simulink library "lib_wheel2"  (Simulink 4.1.1)
values from neighbouring files (symbols this model uses):
  logFlag = 1    [advSACompMaskInit.m]    (also in advSACompMaskInitR13.m)
undefined symbols (not defined in the file or in its folder): lib_help, NOTES, veh_air_density, veh_CD, veh_cg_height, veh_FA, veh_front_wt_frac, veh_gravity, veh_roadwheel_radius, veh_rr_a, veh_rr_alpha, veh_rr_b, veh_rr_beta, veh_rr_c, veh_wheelbase, wh_1st_rrc, wh_2nd_rrc, wh_axle_loss_mass, wh_axle_loss_trq, wh_fa_dl_brake_frac, wh_fa_dl_brake_mph, wh_fa_fric_brake_frac, wh_fa_fric_brake_mph, wh_front_active_bool, wh_inertia, wh_max_front_brake_force, wh_max_rear_brake_force, wh_pressure, wh_radius, wh_rear_active_bool, wh_slip, wh_slip_force_coeff
libraries: lib_wheel2 x61, lib_vehicle x2, lib_etc x2, lib_controls x2, lib_wheel x1
(part 1 of 14)
settings Model: LastModifiedBy=mokeefe
settings Model: ModifiedComment=|
  | mokeefe -- Thu Apr 18 08:40:34 2002 -- Version 1.10
  | saving the model:
  | o "without the model browser open"
  | o with only top-level screen visible
  | o with "fit to view" enabled
  | o with "status bar" off and "toolbar" off
  | o with "prompt to update model history with each save" on
settings Model: ModifiedHistory=|
  | mokeefe -- Thu Apr 18 08:40:34 2002 -- Version 1.10
  | saving the model:
  | o "without the model browser open"
  | o with only top-level screen visible
  | o with "fit to view" enabled
  | o with "status bar" off and "toolbar" off
  | o with "prompt to update model history with each save" on
  | 
  | mokeefe -- Thu Apr 18 08:40:34 2002 -- Version 1.10
  | saving the model:
  | o "without the model browser open"
  | o with only top-level screen visible
  | o with "fit to view" enabled
  | o with "status bar" off and "toolbar" off
  | o with "prompt to update model history with each save" on
  | 
  | ssprik -- Fri Feb 01 16:13:25 2002 -- Version 1.9
  | added wheel goto tag wh_trq_a
  | 
  | mokeefe -- Fri Jun 29 14:51:12 2001 -- Version 1.8
  | 
  | added sub-model component to calculate vehicle weight
  | 
  | mokeefe -- Fri Jun 29 14:49:48 2001 -- Version 1.7
  | 
  | 
  | mokeefe -- Thu Jun 28 14:08:49 2001 -- Version 1.6
  | 
  | replaced all 'veh_mass' references with a veh_mass plus a FROM block (originating from drive cycle) that gives variable cargo mass by time

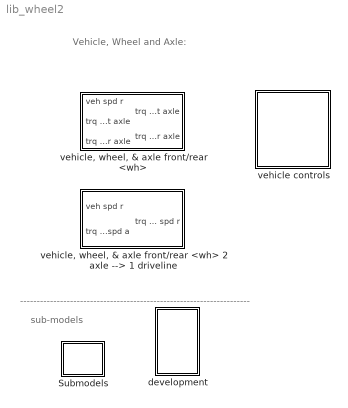
== system lib_wheel2 ==
  note: Vehicle, Wheel and Axle:
  note: ---------------------------------------------------------------------
  note: sub-models
  Submodels : Subsystem
      settings: RTWFcnNameOpts=Auto  RTWFileNameOpts=Auto
  development : Subsystem
      settings: RTWFcnNameOpts=Auto  RTWFileNameOpts=Auto
  vehicle controls : Subsystem
      settings: RTWFcnNameOpts=Auto  RTWFileNameOpts=Auto
  "vehicle, wheel, & axle front/rear <wh>" : Subsystem  mask(Stand-Alone Vehicle, Wheel, & Axle Mask){generalName='veh', generalName01='wh', logPick=Log, initFileName={}, modCell={}, imgFileName='bdi_wh&veh.jpg', DEBUG=OFF}
      mask prompts: generalName "General Name of Vehicle Component [char]"; generalName01 "General Name of Wheel Component [char]"; logPick "Log Variables to Workspace?"; initFileName "Initialization File(s) for VEH and WH [cell array of char]"; modCell "Modification Cell [2 column cell array of param and val]"; imgFileName "Icon image file name [char--evaluated]"
      mask init:
      | % initialization via m-file script
      | advSACompMaskInit;
      settings: RTWFcnNameOpts=Auto  RTWFileNameOpts=Auto
      mask StyleString: edit,edit,popup(Don't Log|Log),edit,edit,edit,popup(ON|OFF)
      mask Display: image(imread(imgFileName))
  "vehicle, wheel, & axle front/rear <wh> 2 axle --> 1 driveline" : Subsystem  mask(Stand-Alone Vehicle, Wheel, & Axle Mask){generalName='veh', generalName01='wh', logPick=Log, initFileName={}, modCell={}, imgFileName='bdi_wh&veh.jpg', DEBUG=OFF}
      mask prompts: generalName "General Name of Vehicle Component [char]"; generalName01 "General Name of Wheel Component [char]"; logPick "Log Variables to Workspace?"; initFileName "Initialization File(s) for VEH and WH [cell array of char]"; modCell "Modification Cell [2 column cell array of param and val]"; imgFileName "Icon image file name [char--evaluated]"
      mask init:
      | % initialization via m-file script
      | advSACompMaskInit;
      settings: RTWFcnNameOpts=Auto  RTWFileNameOpts=Auto
      mask StyleString: edit,edit,popup(Don't Log|Log),edit,edit,edit,popup(ON|OFF)
      mask Display: image(imread(imgFileName))

== system lib_wheel2/Submodels ==
  2 axle --> 1 driveline converter : Subsystem
      settings: RTWFcnNameOpts=Auto  RTWFileNameOpts=Auto
  braking strategy : Subsystem
      settings: RTWFcnNameOpts=Auto  RTWFileNameOpts=Auto
  config traction control : Subsystem  BlockChoice=traction control 2 axle
      settings: TemplateBlock=self  MemberBlocks=traction control 2 axle,traction control J2452 2 axle  RTWFcnNameOpts=Auto  RTWFileNameOpts=Auto
  current veh mass : Subsystem
      settings: RTWFcnNameOpts=Auto  RTWFileNameOpts=Auto
  force req'd to overcome rolling resistance (N) : Subsystem
      settings: RTWFcnNameOpts=Auto  RTWFileNameOpts=Auto
  force req'd to overcome rolling resistance (N) j2452 : Subsystem
      settings: RTWFcnNameOpts=Auto  RTWFileNameOpts=Auto
  front and rear brake controller (achievable) : Subsystem
      settings: RTWFcnNameOpts=Auto  RTWFileNameOpts=Auto
  rolling resistance force : Subsystem  BlockChoice=force req'd to overcome rolling resistance (N)
      settings: TemplateBlock=self  MemberBlocks=force req'd to overcome rolling resistance (N),force req'd to overcome rolling resistance (N) j2452  RTWFcnNameOpts=Auto  RTWFileNameOpts=Auto
  traction control 2 axle : Subsystem
      settings: RTWFcnNameOpts=Auto  RTWFileNameOpts=Auto
  traction control J2452 2 axle : Subsystem
      settings: RTWFcnNameOpts=Auto  RTWFileNameOpts=Auto
  vehicle speed : Subsystem  BlockChoice=vehicle speed (m/s)
      settings: TemplateBlock=self  MemberBlocks=vehicle speed (m/s),vehicle speed (m/s) j2452  RTWFcnNameOpts=Auto  RTWFileNameOpts=Auto
  vehicle speed (m/s) : Subsystem
      settings: RTWFcnNameOpts=Auto  RTWFileNameOpts=Auto
  vehicle speed (m/s) j2452 : Subsystem
      settings: RTWFcnNameOpts=Auto  RTWFileNameOpts=Auto

== system lib_wheel2/development ==
  wheel and axle  front/rear <wh> : Subsystem  mask(Stand-Alone Wheel/Axle Mask){generalName='wh', logPick=Log, initFileName={}, modCell={}, imgFileName='bdi_wh.jpg', DEBUG=OFF}
      mask prompts: generalName "General Name of this Component [char]"; logPick "Log Variables to Workspace?"; initFileName "Initialization File(s) [cell array of char]"; modCell "Modification Cell [2 column cell array of param and val]"; imgFileName "Icon image file name [char--evaluated]"
      mask init:
      | % initialization via m-file script
      | %advSACompMaskInit;
      settings: RTWFcnNameOpts=Auto  RTWFileNameOpts=Auto
      mask StyleString: edit,popup(Don't Log|Log),edit,edit,edit,popup(ON|OFF)
      mask Display: image(imread(imgFileName))
  wheel and axle  front/rear <wh> 2 axle --> 1 driveline : Subsystem
      settings: RTWFcnNameOpts=Auto  RTWFileNameOpts=Auto
      mask Display: image(imread('bdi_wh.jpg'))

== system lib_wheel2/vehicle controls ==
  Bus Selector : BusSelector  OutputSignals=signal1  MuxedOutput=off
  Bus Selector1 : BusSelector  OutputSignals=signal1  MuxedOutput=off
  Bus Selector2 : BusSelector  OutputSignals=signal1  MuxedOutput=off
  dummy controls : Subsystem
      settings: RTWFcnNameOpts=Auto  RTWFileNameOpts=Auto
  tag scope: vehControl=global
  wires:
  dummy controls/1(control sig) -> [vehControl]
  [Sensors] -> Bus Selector/1
  Bus Selector/1 -> dummy controls/1(initial vehicle velocity (m/s))  "<signal1>"
  Bus Selector1/1 -> dummy controls/2(vehicle's current mass (kg))  "<signal1>"
  Bus Selector2/1 -> dummy controls/3(current road grade)  "<signal1>"
  [Sensors] -> Bus Selector2/1
  [Sensors] -> Bus Selector1/1

== system lib_wheel2/vehicle, wheel, & axle front/rear <wh> ==
  note: Vehicle, Wheel, and Axle
  veh spd r : Inport  Port=1  LatchInput=off
  "trq & spd a, front axle" : Inport  Port=2  LatchInput=off
  "trq & spd a, rear axle" : Inport  Port=3  LatchInput=off
  models and interface : Subsystem
      settings: RTWFcnNameOpts=Auto  RTWFileNameOpts=Auto
  "trq & spd r, front axle" : Outport  Port=1  InitialOutput=0
  "trq & spd r, rear axle" : Outport  Port=2  InitialOutput=0
  tag scope: vehReqOut=global, vehSensors=global
  wires:
  veh spd r/1 -> models and interface/1(vehicle speed req'd at end of time step (m/s))
  "trq & spd a, front axle"/1 -> models and interface/2("torque and speed available from drivetrain into front axle (Nm), (rad/s)")
  "trq & spd a, rear axle"/1 -> models and interface/3("torque and speed available from drivetrain into rear axle (Nm), (rad/s)")
  [vehControl] -> models and interface/4(control)
  models and interface/1(requested out) -> [vehReqOut]
  models and interface/2(torque and speed req'd from drivetrain into front axle (Nm),(rad/s)) -> "trq & spd r, front axle"/1
  models and interface/3(torque and speed req'd from drivetrain into rear axle (Nm),(rad/s)) -> "trq & spd r, rear axle"/1
  models and interface/4(sensors) -> [vehSensors]

== system lib_wheel2/vehicle, wheel, & axle front/rear <wh> 2 axle --> 1 driveline ==
  note: Vehicle, Wheel, and Axle
      | 2 axles --> 1 driveline
  veh spd r : Inport  Port=1  LatchInput=off
  trq & spd a : Inport  Port=2  LatchInput=off
  models and interface : Subsystem  AncestorBlock=|
      | lib_wheel2/vehicle, wheel, & axle
      | front//rear <wh>
      | 2 axle --> 1 driveline/models and interface
      settings: RTWFcnNameOpts=Auto  RTWFileNameOpts=Auto
  trq & spd r : Outport  Port=1  InitialOutput=0
  tag scope: vehReqOut=global, vehSensors=global
  wires:
  models and interface/3(sensors) -> [vehSensors]
  models and interface/2(torque and speed req'd from drivetrain into axles (Nm),(rad/s)) -> trq & spd r/1
  models and interface/1(requested out) -> [vehReqOut]
  [vehControl] -> models and interface/3(control)
  trq & spd a/1 -> models and interface/2("torque and speed available from drivetrain into axles (Nm), (rad/s)")
  veh spd r/1 -> models and interface/1(vehicle speed req'd at end of time step (m/s))

== system lib_wheel2/Submodels/2 axle --> 1 driveline converter ==
  front req : Inport  Port=1  LatchInput=off
  rear req : Inport  Port=2  LatchInput=off
  ach : Inport  Port=3  LatchInput=off
  Constant : Constant  Value=wh_front_active_bool
  Constant1 : Constant  Value=wh_rear_active_bool
  Constant2 : Constant  Value=wh_front_active_bool
  Constant3 : Constant  Value=wh_rear_active_bool
  Constant4 : Constant  Value=eps
  Constant5 : Constant  Value=0
  Demux : Demux  Outputs=2  BusSelectionMode=off
  Demux1 : Demux  Outputs=2  BusSelectionMode=off
  Demux2 : Demux  Outputs=2  BusSelectionMode=off
  Ground : Ground
  Logical Operator : Logic  Operator=NAND  Inputs=2
  Mux{,1..3} (4 alike) : Mux  Inputs=2
  Product : Product  Inputs=*/  Multiplication=Element-wise(.*)  SaturateOnIntegerOverflow=on
  Product1 : Product  Inputs=2  Multiplication=Element-wise(.*)  SaturateOnIntegerOverflow=on
  Sum : Sum  Inputs=++  SaturateOnIntegerOverflow=on
  Sum1 : Sum  Inputs=+-  SaturateOnIntegerOverflow=on
  Sum2 : Sum  Inputs=++  SaturateOnIntegerOverflow=on
  Switch{,1..6} (7 alike) : Switch  Threshold=eps
  Terminator : Terminator
  req : Outport  Port=1
  front ach : Outport  Port=2
  rear ach : Outport  Port=3
  wires:
  rear req/1 -> Demux1/1, Switch/3
  Constant/1 -> Switch/2, Logical Operator/1
  Switch/1 -> Switch1/1
  Logical Operator/1 -> Switch1/2, Switch2/2, Switch5/2
  Switch1/1 -> req/1
  Mux/1 -> Switch1/3
  Demux1/1 -> Sum/2
  Demux/1 -> Sum/1, Product/1
  Sum/1 -> Mux/1, Sum2/1, Switch6/2
  Demux/2 -> Mux/2
  Demux1/2 -> Terminator/1
  front req/1 -> Demux/1, Switch/1
  Constant1/1 -> Logical Operator/2
  ach/1 -> Demux2/1, Switch2/1, Switch5/1
  Switch3/1 -> front ach/1
  Switch4/1 -> rear ach/1
  Demux2/1 -> Product1/2, Sum1/1
  Product/1 -> Product1/1
  Sum1/1 -> Mux1/1
  Constant3/1 -> Switch4/2
  Constant2/1 -> Switch3/2
  Ground/1 -> Mux3/1
  Mux3/1 -> Switch4/3, Switch3/3
  Mux2/1 -> Switch2/3
  Mux1/1 -> Switch5/3
  Switch2/1 -> Switch3/1
  Switch5/1 -> Switch4/1
  Demux2/2 -> Mux1/2, Mux2/2, Mux3/2
  Constant4/1 -> Sum2/2
  Sum2/1 -> Product/2
  Product1/1 -> Switch6/1
  Switch6/1 -> Mux2/1, Sum1/2
  Constant5/1 -> Switch6/3

== system lib_wheel2/Submodels/braking strategy ==
  req'd speed (m/s) : Inport  Port=1  LatchInput=off
  slip-limited force req'd (N) : Inport  Port=2  LatchInput=off
  Block NOTES : Subsystem
      settings: RTWFcnNameOpts=Auto  RTWFileNameOpts=Auto
      mask Display: disp('Block\nNOTES')
  Constant : Constant  Orientation=left  Value=0
  Constant1 : Constant  Orientation=left  Value=1
  Constant2 : Constant  Orientation=left  Value=0
  Keep frac>0 : Saturate  UpperLimit=1  LowerLimit=0  LinearizeAsGain=on
  Product : Product  Inputs=2  Multiplication=Element-wise(.*)  SaturateOnIntegerOverflow=on
  Product1 : Product  Inputs=2  Multiplication=Element-wise(.*)  SaturateOnIntegerOverflow=on
  Sum : Sum  Inputs=--+  SaturateOnIntegerOverflow=on
  Switch : Switch  Threshold=0
  Switch1 : Switch  Threshold=0
  convert (mph) : Gain  Gain=2.2371  Multiplication=Element-wise(K.*u)  SaturateOnIntegerOverflow=on
  front driveline braking fraction : Lookup  InputValues=wh_fa_dl_brake_mph  OutputValues=wh_fa_dl_brake_frac
  front friction braking fraction : Lookup  InputValues=wh_fa_fric_brake_mph  OutputValues=wh_fa_fric_brake_frac
  req'd front brake force (N) : Outport  Port=1  InitialOutput=0
  req'd rear brake force (N) : Outport  Port=2  InitialOutput=0
  wires:
  Keep frac>0/1 -> Product1/2
  Sum/1 -> Keep frac>0/1
  Constant/1 -> Switch/1
  Product/1 -> Switch/3
  slip-limited force req'd (N)/1 -> Switch/2, Product/1, Product1/1, Switch1/2
  Switch/1 -> req'd front brake force (N)/1
  Product1/1 -> Switch1/3
  Constant2/1 -> Switch1/1
  Switch1/1 -> req'd rear brake force (N)/1
  req'd speed (m/s)/1 -> convert (mph)/1
  convert (mph)/1 -> front friction braking fraction/1, front driveline braking fraction/1
  front driveline braking fraction/1 -> Sum/2
  front friction braking fraction/1 -> Product/2, Sum/1
  Constant1/1 -> Sum/3

== system lib_wheel2/Submodels/config traction control ==
  time-average vehicle speed  req'd (m/s) : Inport  Port=1  LatchInput=off
  vehicle speed at beginning of time  step (m/s) : Inport  Port=2  LatchInput=off
  total tractive force req'd (N) : Inport  Port=3  LatchInput=off
  traction control 2 axle : Subsystem
      settings: RTWFcnNameOpts=Auto  RTWFileNameOpts=Auto
  req'd force (N) : Outport  Port=1
  req'd speed (m/s) : Outport  Port=2
  weight on front axle (N) : Outport  Port=3
  weight on rear axle (N) : Outport  Port=4
  front/total  traction ratio : Outport  Port=5
  wires:
  time-average vehicle speed  req'd (m/s)/1 -> ?
  vehicle speed at beginning of time  step (m/s)/1 -> ?
  total tractive force req'd (N)/1 -> ?
  ? -> req'd force (N)/1
  ? -> req'd speed (m/s)/1
  ? -> weight on front axle (N)/1
  ? -> weight on rear axle (N)/1
  ? -> front/total  traction ratio/1

== system lib_wheel2/Submodels/current veh mass ==
  current veh mass (kg) : Outport  Port=1
  wires:
  [current_veh_mass] -> current veh mass (kg)/1

== system lib_wheel2/Submodels/force req'd to overcome rolling resistance (N) ==
  average vehicle speed over time step (m/s) : Inport  Port=1  LatchInput=off
  Constant : Constant  Value=wh_1st_rrc
  Constant1 : Constant  Orientation=up  Value=0
  Constant2 : Constant  Orientation=left  Value=veh_gravity
  Gain1 : Gain  Gain=wh_2nd_rrc  Multiplication=Element-wise(K.*u)  SaturateOnIntegerOverflow=on
  Product : Product  Inputs=4  Multiplication=Element-wise(.*)  SaturateOnIntegerOverflow=on
  Sum : Sum  Inputs=++  SaturateOnIntegerOverflow=on
  Switch : Switch  Threshold=eps
  Trig Fn2 : Trigonometry  Operator=atan  OutputSignalType=auto
  Trig Fn3 : Trigonometry  Operator=cos  OutputSignalType=auto
  current veh mass : lib_wheel2/Submodels/current veh mass
      settings: RTWFcnNameOpts=Auto  RTWFileNameOpts=Auto
  Fr (N) : Outport  Port=1  InitialOutput=0
  wires:
  Trig Fn2/1 -> Trig Fn3/1
  [grade] -> Trig Fn2/1
  current veh mass/1 -> Product/4
  Trig Fn3/1 -> Product/3
  Product/1 -> Switch/1
  Constant2/1 -> Product/1
  Sum/1 -> Product/2
  Constant1/1 -> Switch/3
  average vehicle speed over time step (m/s)/1 -> Switch/2, Gain1/1
  Switch/1 -> Fr (N)/1
  Gain1/1 -> Sum/2
  Constant/1 -> Sum/1

== system lib_wheel2/Submodels/force req'd to overcome rolling resistance (N) j2452 ==
  average vehicle speed over time step (m/s) : Inport  Port=1  LatchInput=off
  Constant1 : Constant  Orientation=up  Value=0
  Constant2 : Constant  Value=veh_gravity
  Constant3 : Constant  Value=veh_rr_beta
  Constant4 : Constant  Value=wh_pressure
  Constant5 : Constant  Value=veh_rr_alpha
  Constant6 : Constant  Value=veh_rr_a
  Constant7 : Constant  Value=veh_front_wt_frac
  Constant8 : Constant  Value=0.5
  Constant9 : Constant  Value=1
  Convert (m/s) to (km/h) : Gain  Description=Conversion of m/s to km/h  Gain=3.6  Multiplication=Element-wise(K.*u)  SaturateOnIntegerOverflow=on
  Curvature Correction Factor : Constant  Value=(veh_roadwheel_radius/(veh_roadwheel_radius+wh_radius))
  Gain : Gain  Gain=veh_rr_b  Multiplication=Element-wise(K.*u)  SaturateOnIntegerOverflow=on
  Gain1 : Gain  Gain=2  Multiplication=Element-wise(K.*u)  SaturateOnIntegerOverflow=on
  Gain2 : Gain  Gain=veh_rr_c  Multiplication=Element-wise(K.*u)  SaturateOnIntegerOverflow=on
  Gain3 : Gain  Gain=2  Multiplication=Element-wise(K.*u)  SaturateOnIntegerOverflow=on
  Math Function : Math  Operator=pow  OutputSignalType=auto
  Math Function1 : Math  Operator=pow  OutputSignalType=auto
  Math Function2 : Math  Operator=pow  OutputSignalType=auto
  Math Function3 : Math  Operator=sqrt  OutputSignalType=auto
  NOTES : Subsystem  Description=Notes  Orientation=left  AncestorBlock=lib_help/NOTES
      settings: RTWFcnNameOpts=Auto  RTWFileNameOpts=Auto
      mask Display: disp('Block\nNOTES')
  Product : Product  Inputs=3  Multiplication=Element-wise(.*)  SaturateOnIntegerOverflow=on
  Product2 : Product  Inputs=4  Multiplication=Element-wise(.*)  SaturateOnIntegerOverflow=on
  Product3 : Product  Inputs=3  Multiplication=Element-wise(.*)  SaturateOnIntegerOverflow=on
  Product4 : Product  Inputs=3  Multiplication=Element-wise(.*)  SaturateOnIntegerOverflow=on
  Squaring Function : Math  Operator=square  OutputSignalType=auto
  Sum1 : Sum  Inputs=++  SaturateOnIntegerOverflow=on
  Sum2 : Sum  Inputs=+++  SaturateOnIntegerOverflow=on
  Sum3 : Sum  Inputs=-+  SaturateOnIntegerOverflow=on
  Switch : Switch  Threshold=eps
  Trig Fn2 : Trigonometry  Operator=atan  OutputSignalType=auto
  Trig Fn3 : Trigonometry  Operator=cos  OutputSignalType=auto
  current veh mass : lib_wheel2/Submodels/current veh mass
      settings: RTWFcnNameOpts=Auto  RTWFileNameOpts=Auto
  Fr (N) : Outport  Port=1  InitialOutput=0
  wires:
  Curvature Correction Factor/1 -> Math Function3/1
  Math Function3/1 -> Product2/4
  Constant3/1 -> Math Function2/2, Math Function/2
  Convert (m/s) to (km/h)/1 -> Switch/2, Gain/1, Squaring Function/1
  average vehicle speed over time step (m/s)/1 -> Convert (m/s) to (km/h)/1
  Constant5/1 -> Math Function1/2
  Sum2/1 -> Product2/1
  Sum1/1 -> Product2/2
  Math Function1/1 -> Product2/3
  Gain3/1 -> Sum1/2
  Math Function2/1 -> Gain3/1
  Product4/1 -> Math Function2/1
  Sum3/1 -> Product4/3
  Constant9/1 -> Sum3/2
  Gain1/1 -> Sum1/1
  Product3/1 -> Math Function/1
  Constant8/1 -> Product4/2, Product3/3
  Constant7/1 -> Sum3/1, Product3/2
  Product/1 -> Product4/1, Product3/1
  Switch/1 -> Fr (N)/1
  Product2/1 -> Switch/1
  Gain2/1 -> Sum2/3
  Gain/1 -> Sum2/2
  Constant6/1 -> Sum2/1
  Squaring Function/1 -> Gain2/1
  Math Function/1 -> Gain1/1
  Constant4/1 -> Math Function1/1
  current veh mass/1 -> Product/3
  Constant2/1 -> Product/2
  Trig Fn3/1 -> Product/1
  [grade] -> Trig Fn2/1
  Constant1/1 -> Switch/3
  Trig Fn2/1 -> Trig Fn3/1

== system lib_wheel2/Submodels/front and rear brake controller (achievable) ==
  total tractive force req'd (N) : Inport  Port=1  LatchInput=off
  tractive force available from  front drivetrain (N) : Inport  Port=2  LatchInput=off
  axle speed possible (rad/s) : Inport  Port=3  LatchInput=off
  max front brake force (N) : Inport  Port=4  LatchInput=off
  max rear brake force (N) : Inport  Port=5  LatchInput=off
  tractive force available from  rear drivetrain (N) : Inport  Port=6  LatchInput=off
  Block NOTES : Subsystem
      settings: RTWFcnNameOpts=Auto  RTWFileNameOpts=Auto
      mask Display: disp('Block\nNOTES')
  Constant : Constant  Orientation=down  Value=0
  Constant1 : Constant  Orientation=down  Value=0
  MinMax : MinMax  Function=min  Inputs=2
  MinMax1 : MinMax  Function=min  Inputs=2
  MinMax2 : MinMax  Function=max  Inputs=2
  Sum1 : Sum  Inputs=+--  SaturateOnIntegerOverflow=on
  Sum2 : Sum  Inputs=+-  SaturateOnIntegerOverflow=on
  Switch: braking force to be split between friction brakes (N) : Switch  Threshold=0
  braking force supplied by front friction brakes (N) : Subsystem
      settings: RTWFcnNameOpts=Auto  RTWFileNameOpts=Auto
  "m/s -> mph (mph)" : Gain  Gain=2.237  Multiplication=Element-wise(K.*u)  SaturateOnIntegerOverflow=on
  "rad/s -> m/s (m/s)" : Gain  Gain=wh_radius  Multiplication=Element-wise(K.*u)  SaturateOnIntegerOverflow=on
  rear braking force req'd (N) : Switch  Threshold=0
  front-axle braking force (N) : Outport  Port=1  InitialOutput=0
  rear-axle braking force (N) : Outport  Port=2  InitialOutput=0
  wires:
  max rear brake force (N)/1 -> MinMax2/2
  max front brake force (N)/1 -> braking force supplied by front friction brakes (N)/3(max front brake force (N))
  Constant1/1 -> rear braking force req'd (N)/1, MinMax/1
  MinMax/1 -> rear braking force req'd (N)/3
  Sum2/1 -> MinMax/2
  rear braking force req'd (N)/1 -> MinMax2/1
  MinMax2/1 -> rear-axle braking force (N)/1
  "rad/s -> m/s (m/s)"/1 -> "m/s -> mph (mph)"/1
  axle speed possible (rad/s)/1 -> "rad/s -> m/s (m/s)"/1
  tractive force available from  front drivetrain (N)/1 -> Sum1/2
  total tractive force req'd (N)/1 -> Sum1/1, Switch: braking force to be split between friction brakes (N)/2
  Sum1/1 -> MinMax1/2
  MinMax1/1 -> Switch: braking force to be split between friction brakes (N)/3
  Constant/1 -> Switch: braking force to be split between friction brakes (N)/1, MinMax1/1
  "m/s -> mph (mph)"/1 -> braking force supplied by front friction brakes (N)/2(possible speed (mph))
  Switch: braking force to be split between friction brakes (N)/1 -> braking force supplied by front friction brakes (N)/1(add'l braking force req'd (N)), rear braking force req'd (N)/2, Sum2/1
  braking force supplied by front friction brakes (N)/1(braking force from front-axle friction brakes (N)) -> Sum2/2, front-axle braking force (N)/1
  tractive force available from  rear drivetrain (N)/1 -> Sum1/3

== system lib_wheel2/Submodels/rolling resistance force ==
  average vehicle speed over time step (m/s) : Inport  Port=1  LatchInput=off
  force req'd to overcome rolling resistance (N) : lib_vehicle/Submodels/force req'd to overcome rolling resistance (N)
      settings: RTWFcnNameOpts=Auto  RTWFileNameOpts=Auto
  Fr (N) : Outport  Port=1
  wires:
  average vehicle speed over time step (m/s)/1 -> force req'd to overcome rolling resistance (N)/1
  force req'd to overcome rolling resistance (N)/1 -> Fr (N)/1

== system lib_wheel2/Submodels/traction control 2 axle ==
  time-average vehicle speed  req'd (m/s) : Inport  Port=1  LatchInput=off
  vehicle speed at beginning of time  step (m/s) : Inport  Port=2  LatchInput=off
  total tractive force req'd (N) : Inport  Port=3  LatchInput=off
  Block NOTES : Subsystem
      settings: RTWFcnNameOpts=Auto  RTWFileNameOpts=Auto
      mask Display: disp('Block\nNOTES')
  apply tire traction limit to req'd speed (m/s) : Subsystem
      settings: RTWFcnNameOpts=Auto  RTWFileNameOpts=Auto
  enforce max.  front axle tractive force  due to slip (N) : Subsystem
      settings: RTWFcnNameOpts=Auto  RTWFileNameOpts=Auto
  req'd force (N) : Outport  Port=1  InitialOutput=0
  req'd speed (m/s) : Outport  Port=2  InitialOutput=0
  weight on front axle (N) : Outport  Port=3  InitialOutput=0
  weight on rear axle (N) : Outport  Port=4  InitialOutput=0
  front/total  traction ratio : Outport  Port=5  InitialOutput=0
  wires:
  apply tire traction limit to req'd speed (m/s)/1(out_1) -> enforce max.  front axle tractive force  due to slip (N)/2(requested time-step average vehicle speed (m/s)), req'd speed (m/s)/1
  total tractive force req'd (N)/1 -> enforce max.  front axle tractive force  due to slip (N)/1(tractive force req'd at tire/road interface (N))
  enforce max.  front axle tractive force  due to slip (N)/1(slip-limited force (N)) -> req'd force (N)/1
  enforce max.  front axle tractive force  due to slip (N)/2(weight on front axle (N)) -> weight on front axle (N)/1
  vehicle speed at beginning of time  step (m/s)/1 -> enforce max.  front axle tractive force  due to slip (N)/3(speed at beginning of time step (m/s)), apply tire traction limit to req'd speed (m/s)/2(vehicle speed at beginning of time step (m/s))
  time-average vehicle speed  req'd (m/s)/1 -> apply tire traction limit to req'd speed (m/s)/1("requested time-step  average vehicle speed (m/s) ")
  enforce max.  front axle tractive force  due to slip (N)/3(weight on rear axle (N)) -> weight on rear axle (N)/1
  enforce max.  front axle tractive force  due to slip (N)/4(front/total traction ratio) -> front/total  traction ratio/1

== system lib_wheel2/Submodels/traction control J2452 2 axle ==
  time-average vehicle speed  req'd (m/s) : Inport  Port=1  LatchInput=off
  vehicle speed at beginning of time  step (m/s) : Inport  Port=2  LatchInput=off
  total tractive force req'd (N) : Inport  Port=3  LatchInput=off
  Block NOTES : Subsystem
      settings: RTWFcnNameOpts=Auto  RTWFileNameOpts=Auto
      mask Display: disp('Block\nNOTES')
  apply tire traction limit to req'd speed (m/s) : Subsystem
      settings: RTWFcnNameOpts=Auto  RTWFileNameOpts=Auto
  enforce max.  front axle tractive force  due to slip (N) : lib_wheel2/Submodels/traction control 2 axle/enforce max.  front axle tractive force  due to slip (N)
      settings: RTWFcnNameOpts=Auto  RTWFileNameOpts=Auto
  req'd force (N) : Outport  Port=1  InitialOutput=0
  req'd speed (m/s) : Outport  Port=2  InitialOutput=0
  weight on front axle (N) : Outport  Port=3  InitialOutput=0
  weight on rear axle (N) : Outport  Port=4  InitialOutput=0
  front/total  traction ratio : Outport  Port=5  InitialOutput=0
  wires:
  apply tire traction limit to req'd speed (m/s)/1(out_1) -> req'd speed (m/s)/1, enforce max.  front axle tractive force  due to slip (N)/2
  total tractive force req'd (N)/1 -> enforce max.  front axle tractive force  due to slip (N)/1
  enforce max.  front axle tractive force  due to slip (N)/1 -> req'd force (N)/1
  enforce max.  front axle tractive force  due to slip (N)/2 -> weight on front axle (N)/1
  vehicle speed at beginning of time  step (m/s)/1 -> apply tire traction limit to req'd speed (m/s)/2(vehicle speed at beginning of time step (m/s)), enforce max.  front axle tractive force  due to slip (N)/3
  time-average vehicle speed  req'd (m/s)/1 -> apply tire traction limit to req'd speed (m/s)/1("requested time-step  average vehicle speed (m/s) ")
  enforce max.  front axle tractive force  due to slip (N)/3 -> weight on rear axle (N)/1
  enforce max.  front axle tractive force  due to slip (N)/4 -> front/total  traction ratio/1

== system lib_wheel2/Submodels/vehicle speed ==
  vehicle speed at beginning of time step (m/s) : Inport  Port=1  LatchInput=off
  "available tractive force and linear speed (N), (m/s)" : Inport  Port=2  LatchInput=off
  vehicle speed (m/s) : lib_vehicle/Submodels/vehicle speed (m//s)
      settings: RTWFcnNameOpts=Auto  RTWFileNameOpts=Auto
  vehicle speed achievable at end of time step (m/s) : Outport  Port=1
  wires:
  vehicle speed at beginning of time step (m/s)/1 -> vehicle speed (m/s)/1
  "available tractive force and linear speed (N), (m/s)"/1 -> vehicle speed (m/s)/2
  vehicle speed (m/s)/1 -> vehicle speed achievable at end of time step (m/s)/1

== system lib_wheel2/Submodels/vehicle speed (m/s) ==
  vehicle speed at beginning of time step (m/s) : Inport  Port=1  LatchInput=off
  "available tractive force and linear speed (N), (m/s)" : Inport  Port=2  LatchInput=off
  Block NOTES : Subsystem
      settings: RTWFcnNameOpts=Auto  RTWFileNameOpts=Auto
      mask Display: disp('Block\nNOTES')
  Clock : Clock
      settings: DisplayTime=off  Decimation=10
  Constant : Constant  Orientation=left  Value=0
  Demux : Demux  Outputs=2  BusSelectionMode=off
  Gain : Gain  Gain=-1  Multiplication=Element-wise(K.*u)  SaturateOnIntegerOverflow=on
  Gain1 : Gain  Gain=2  Multiplication=Element-wise(K.*u)  SaturateOnIntegerOverflow=on
  Memory : Memory  X0=-.1  InheritSampleTime=off
      settings: RTWStateStorageClass=Auto
  MinMax : MinMax  Function=min  Inputs=2
  MinMax1 : MinMax  Function=max  Inputs=2
  Mux : Mux  Inputs=3
      settings: DisplayOption=none
  Relational Operator : RelationalOperator  Operator=>=
  Sum5 : Sum  Inputs=-+  SaturateOnIntegerOverflow=on
  Switch : Switch  Threshold=0.5
  Switch1 : Switch  Threshold=1e-9
  Trig Fn4 : Trigonometry  Operator=atan  OutputSignalType=auto
  a : Constant  Value=0.5*veh_air_density*veh_CD*veh_FA
  b : Subsystem
      settings: RTWFcnNameOpts=Auto  RTWFileNameOpts=Auto
  c : Subsystem
      settings: RTWFcnNameOpts=Auto  RTWFileNameOpts=Auto
  current veh mass1 : lib_wheel2/Submodels/current veh mass
      settings: RTWFcnNameOpts=Auto  RTWFileNameOpts=Auto
  dt : Sum  Inputs=+-  SaturateOnIntegerOverflow=on
  only have rolling resistance if moving : Fcn  Expr=u>0
  solve the quadratic for avg. linear spd : Fcn  Expr=(-u[2]+(u[2]^2-4*u[1]*u[3])^.5)/(2*u[1])
  vehicle speed achievable at end of time step (m/s) : Outport  Port=1  InitialOutput=0
  wires:
  Relational Operator/1 -> Switch/2
  current veh mass1/1 -> Gain/1
  Gain/1 -> Relational Operator/2
  Switch/1 -> Gain1/1
  solve the quadratic for avg. linear spd/1 -> MinMax/1, MinMax1/1
  Gain1/1 -> Sum5/2
  MinMax1/1 -> Switch/3
  MinMax/1 -> Switch/1
  a/1 -> Mux/1
  Mux/1 -> solve the quadratic for avg. linear spd/1
  Switch1/1 -> vehicle speed achievable at end of time step (m/s)/1
  b/1(b) -> Mux/2
  Clock/1 -> dt/1, Memory/1
  Memory/1 -> dt/2
  [grade] -> Trig Fn4/1
  dt/1 -> b/1(dt), c/1(dt)
  Trig Fn4/1 -> b/2(angle of elevation), c/4(angle of elevation)
  only have rolling resistance if moving/1 -> b/3(vehicle moving?), c/5(vehicle moving?)
  Sum5/1 -> Switch1/1, Switch1/2
  Constant/1 -> Switch1/3
  "available tractive force and linear speed (N), (m/s)"/1 -> Demux/1
  c/1(c) -> Mux/3
  Demux/2 -> only have rolling resistance if moving/1, MinMax/2, MinMax1/2
  Demux/1 -> Relational Operator/1, c/3(Ftract)
  vehicle speed at beginning of time step (m/s)/1 -> c/2(v_prev), Sum5/1

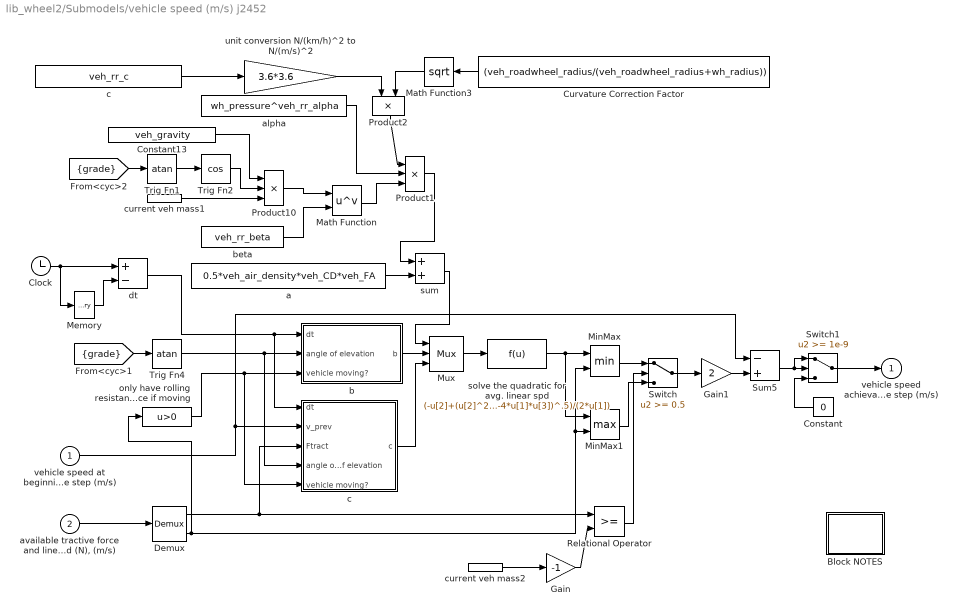
== system lib_wheel2/Submodels/vehicle speed (m/s) j2452 ==
  vehicle speed at beginning of time step (m/s) : Inport  Port=1  LatchInput=off
  "available tractive force and linear speed (N), (m/s)" : Inport  Port=2  LatchInput=off
  Block NOTES : Subsystem
      settings: RTWFcnNameOpts=Auto  RTWFileNameOpts=Auto
      mask Display: disp('Block\nNOTES')
  Clock : Clock
      settings: DisplayTime=off  Decimation=10
  Constant : Constant  Orientation=left  Value=0
  Constant13 : Constant  Value=veh_gravity
  Curvature Correction Factor : Constant  Orientation=left  Value=(veh_roadwheel_radius/(veh_roadwheel_radius+wh_radius))  VectorParams1D=off
  Demux : Demux  Outputs=2  BusSelectionMode=off
  Gain : Gain  Gain=-1  Multiplication=Element-wise(K.*u)  SaturateOnIntegerOverflow=on
  Gain1 : Gain  Gain=2  Multiplication=Element-wise(K.*u)  SaturateOnIntegerOverflow=on
  Math Function : Math  Operator=pow  OutputSignalType=auto
  Math Function3 : Math  Orientation=left  Operator=sqrt  OutputSignalType=auto
  Memory : Memory  X0=-.1  InheritSampleTime=off
      settings: RTWStateStorageClass=Auto
  MinMax : MinMax  Function=min  Inputs=2
  MinMax1 : MinMax  Function=max  Inputs=2
  Mux : Mux  Inputs=3
      settings: DisplayOption=none
  Product1 : Product  Inputs=3  Multiplication=Element-wise(.*)  SaturateOnIntegerOverflow=on
  Product10 : Product  Inputs=3  Multiplication=Element-wise(.*)  SaturateOnIntegerOverflow=on
  Product2 : Product  Orientation=down  Inputs=2  Multiplication=Element-wise(.*)  SaturateOnIntegerOverflow=on
  Relational Operator : RelationalOperator  Operator=>=
  Sum5 : Sum  Inputs=-+  SaturateOnIntegerOverflow=on
  Switch : Switch  Threshold=0.5
  Switch1 : Switch  Threshold=1e-9
  Trig Fn1 : Trigonometry  Operator=atan  OutputSignalType=auto
  Trig Fn2 : Trigonometry  Operator=cos  OutputSignalType=auto
  Trig Fn4 : Trigonometry  Operator=atan  OutputSignalType=auto
  a : Constant  Value=0.5*veh_air_density*veh_CD*veh_FA
  alpha : Constant  Value=wh_pressure^veh_rr_alpha
  b : Subsystem
      settings: RTWFcnNameOpts=Auto  RTWFileNameOpts=Auto
  beta : Constant  Value=veh_rr_beta
  c : Subsystem
      settings: RTWFcnNameOpts=Auto  RTWFileNameOpts=Auto
  "c " : Constant  Value=veh_rr_c
  current veh mass1 : lib_wheel2/Submodels/current veh mass
      settings: RTWFcnNameOpts=Auto  RTWFileNameOpts=Auto
  current veh mass2 : lib_wheel2/Submodels/current veh mass
      settings: RTWFcnNameOpts=Auto  RTWFileNameOpts=Auto
  dt : Sum  Inputs=+-  SaturateOnIntegerOverflow=on
  only have rolling resistance if moving : Fcn  Expr=u>0
  solve the quadratic for avg. linear spd : Fcn  Expr=(-u[2]+(u[2]^2-4*u[1]*u[3])^.5)/(2*u[1])
  sum : Sum  Inputs=++  SaturateOnIntegerOverflow=on
  unit conversion N/(km/h)^2 to N/(m/s)^2 : Gain  Gain=3.6*3.6  Multiplication=Element-wise(K.*u)  SaturateOnIntegerOverflow=on
  vehicle speed achievable at end of time step (m/s) : Outport  Port=1  InitialOutput=0
  wires:
  Product2/1 -> Product1/1
  Math Function3/1 -> Product2/2
  unit conversion N/(km/h)^2 to N/(m/s)^2/1 -> Product2/1
  Curvature Correction Factor/1 -> Math Function3/1
  current veh mass1/1 -> Product10/3
  Trig Fn2/1 -> Product10/2
  Constant13/1 -> Product10/1
  Product1/1 -> sum/1
  Math Function/1 -> Product1/3
  alpha/1 -> Product1/2
  "c "/1 -> unit conversion N/(km/h)^2 to N/(m/s)^2/1
  sum/1 -> Mux/1
  a/1 -> sum/2
  beta/1 -> Math Function/2
  Product10/1 -> Math Function/1
  Trig Fn1/1 -> Trig Fn2/1
  [grade] -> Trig Fn1/1
  vehicle speed at beginning of time step (m/s)/1 -> c/2(v_prev), Sum5/1
  Demux/1 -> c/3(Ftract), Relational Operator/1
  Demux/2 -> MinMax1/2, MinMax/2, only have rolling resistance if moving/1
  c/1(c) -> Mux/3
  "available tractive force and linear speed (N), (m/s)"/1 -> Demux/1
  Constant/1 -> Switch1/3
  Sum5/1 -> Switch1/2, Switch1/1
  only have rolling resistance if moving/1 -> c/5(vehicle moving?), b/3(vehicle moving?)
  Trig Fn4/1 -> c/4(angle of elevation), b/2(angle of elevation)
  dt/1 -> c/1(dt), b/1(dt)
  [grade] -> Trig Fn4/1
  Memory/1 -> dt/2
  Clock/1 -> Memory/1, dt/1
  b/1(b) -> Mux/2
  Switch1/1 -> vehicle speed achievable at end of time step (m/s)/1
  Mux/1 -> solve the quadratic for avg. linear spd/1
  MinMax/1 -> Switch/1
  MinMax1/1 -> Switch/3
  Gain1/1 -> Sum5/2
  solve the quadratic for avg. linear spd/1 -> MinMax1/1, MinMax/1
  Switch/1 -> Gain1/1
  Gain/1 -> Relational Operator/2
  current veh mass2/1 -> Gain/1
  Relational Operator/1 -> Switch/2

== system lib_wheel2/development/wheel and axle  front/rear <wh> ==
  note: Wheel and Axle
  "tractive force and speed req'd of tire/road interface (N), (m/s)" : Inport  Port=1  LatchInput=off
  "torque and speed available from drivetrain into front axle (Nm), (rad/s)" : Inport  Port=2  LatchInput=off
  "torque and speed available from drivetrain into rear axle (Nm), (rad/s)" : Inport  Port=3  LatchInput=off
  wheel & axle model & interface : Subsystem
      settings: RTWFcnNameOpts=Auto  RTWFileNameOpts=Auto
  torque and speed req'd from drivetrain into front axle (Nm),(rad/s) : Outport  Port=1  InitialOutput=0
  torque and speed req'd from drivetrain into rear axle (Nm),(rad/s) : Outport  Port=2  InitialOutput=0
  tractive force and linear speed  achievable : Outport  Port=3  InitialOutput=0
  tag scope: whReqOut=global, whSensors=global
  wires:
  wheel & axle model & interface/2(torque and speed req'd from drivetrain into front axle (Nm),(rad/s)) -> torque and speed req'd from drivetrain into front axle (Nm),(rad/s)/1
  "tractive force and speed req'd of tire/road interface (N), (m/s)"/1 -> wheel & axle model & interface/1("tractive force and speed req'd of tire/road interface (N), (m/s)")
  wheel & axle model & interface/3(torque and speed req'd from drivetrain into rear axle (Nm),(rad/s)) -> torque and speed req'd from drivetrain into rear axle (Nm),(rad/s)/1
  "torque and speed available from drivetrain into front axle (Nm), (rad/s)"/1 -> wheel & axle model & interface/2("torque and speed available from drivetrain into front axle (Nm), (rad/s)")
  wheel & axle model & interface/4(tractive force and linear speed  achievable) -> tractive force and linear speed  achievable/1
  "torque and speed available from drivetrain into rear axle (Nm), (rad/s)"/1 -> wheel & axle model & interface/3("torque and speed available from drivetrain into rear axle (Nm), (rad/s)")
  wheel & axle model & interface/1(req out) -> [whReqOut]
  [whControl] -> wheel & axle model & interface/4(control)
  wheel & axle model & interface/5(sensors) -> [whSensors]

== system lib_wheel2/development/wheel and axle  front/rear <wh> 2 axle --> 1 driveline ==
  note: Wheel and Axle
  "tractive force and speed req'd of tire/road interface (N), (m/s)" : Inport  Port=1  LatchInput=off
  "torque and speed available from drivetrain into axle set (Nm), (rad/s)" : Inport  Port=2  LatchInput=off
  wheel & axle model & interface : Subsystem
      settings: RTWFcnNameOpts=Auto  RTWFileNameOpts=Auto
  torque and speed req'd from drivetrain into axle set (Nm),(rad/s) : Outport  Port=1  InitialOutput=0
  tractive force and linear speed  achievable : Outport  Port=2  InitialOutput=0
  tag scope: fcReqOut=global, fcSensors=global
  wires:
  "tractive force and speed req'd of tire/road interface (N), (m/s)"/1 -> wheel & axle model & interface/1("tractive force and speed req'd of tire/road interface (N), (m/s)")
  "torque and speed available from drivetrain into axle set (Nm), (rad/s)"/1 -> wheel & axle model & interface/2("torque and speed available from drivetrain into axle (Nm), (rad/s)")
  [fcControl] -> wheel & axle model & interface/3(control)
  wheel & axle model & interface/1(req out) -> [fcReqOut]
  wheel & axle model & interface/2(sensors) -> torque and speed req'd from drivetrain into axle set (Nm),(rad/s)/1
  wheel & axle model & interface/3(tractive force and linear speed  achievable) -> tractive force and linear speed  achievable/1
  wheel & axle model & interface/4(trq and spd into axle set required) -> [fcSensors]

== system lib_wheel2/vehicle controls/dummy controls ==
  initial vehicle velocity (m/s) : Inport  Port=1  LatchInput=off
  vehicle's current mass (kg) : Inport  Port=2  LatchInput=off
  current road grade : Inport  Port=3  LatchInput=off
  Bus Creator : BusCreator  Inputs=3
  control sig : Outport  Port=1
  wires:
  Bus Creator/1 -> control sig/1
  [grade] -> Bus Creator/3  "grade"
  [current_veh_mass] -> Bus Creator/2  "current_veh_mass"
  [v_init] -> Bus Creator/1  "v_init"
  current road grade/1 -> [grade]
  vehicle's current mass (kg)/1 -> [current_veh_mass]
  initial vehicle velocity (m/s)/1 -> [v_init]

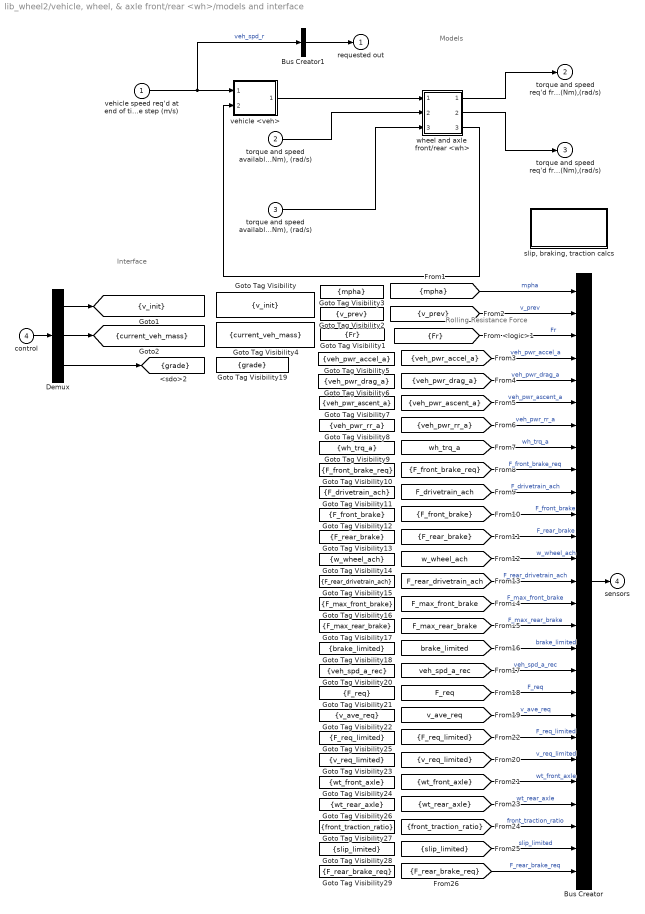
== system lib_wheel2/vehicle, wheel, & axle front/rear <wh>/models and interface ==
  note: Rolling Resistance Force
  note: Models
  note: Interface
  vehicle speed req'd at end of time step (m/s) : Inport  Port=1  LatchInput=off
  "torque and speed available from drivetrain into front axle (Nm), (rad/s)" : Inport  Port=2  LatchInput=off
  "torque and speed available from drivetrain into rear axle (Nm), (rad/s)" : Inport  Port=3  LatchInput=off
  control : Inport  Port=4  LatchInput=off
  Bus Creator : BusCreator  Inputs=27
  Bus Creator1 : BusCreator  Inputs=1
  Demux : Demux  Outputs=3  BusSelectionMode=off
  Goto Tag Visibility : GotoTagVisibility  GotoTag=v_init
  Goto Tag Visibility1 : GotoTagVisibility  GotoTag=Fr
  Goto Tag Visibility10 : GotoTagVisibility  GotoTag=F_front_brake_req
  Goto Tag Visibility11 : GotoTagVisibility  GotoTag=F_drivetrain_ach
  Goto Tag Visibility12 : GotoTagVisibility  GotoTag=F_front_brake
  Goto Tag Visibility13 : GotoTagVisibility  GotoTag=F_rear_brake
  Goto Tag Visibility14 : GotoTagVisibility  GotoTag=w_wheel_ach
  Goto Tag Visibility15 : GotoTagVisibility  GotoTag=F_rear_drivetrain_ach
  Goto Tag Visibility16 : GotoTagVisibility  GotoTag=F_max_front_brake
  Goto Tag Visibility17 : GotoTagVisibility  GotoTag=F_max_rear_brake
  Goto Tag Visibility18 : GotoTagVisibility  GotoTag=brake_limited
  Goto Tag Visibility19 : GotoTagVisibility  GotoTag=grade
  Goto Tag Visibility2 : GotoTagVisibility  GotoTag=v_prev
  Goto Tag Visibility20 : GotoTagVisibility  GotoTag=veh_spd_a_rec
  Goto Tag Visibility21 : GotoTagVisibility  GotoTag=F_req
  Goto Tag Visibility22 : GotoTagVisibility  GotoTag=v_ave_req
  Goto Tag Visibility23 : GotoTagVisibility  GotoTag=v_req_limited
  Goto Tag Visibility24 : GotoTagVisibility  GotoTag=wt_front_axle
  Goto Tag Visibility25 : GotoTagVisibility  GotoTag=F_req_limited
  Goto Tag Visibility26 : GotoTagVisibility  GotoTag=wt_rear_axle
  Goto Tag Visibility27 : GotoTagVisibility  GotoTag=front_traction_ratio
  Goto Tag Visibility28 : GotoTagVisibility  GotoTag=slip_limited
  Goto Tag Visibility29 : GotoTagVisibility  GotoTag=F_rear_brake_req
  Goto Tag Visibility3 : GotoTagVisibility  GotoTag=mpha
  Goto Tag Visibility4 : GotoTagVisibility  GotoTag=current_veh_mass
  Goto Tag Visibility5 : GotoTagVisibility  GotoTag=veh_pwr_accel_a
  Goto Tag Visibility6 : GotoTagVisibility  GotoTag=veh_pwr_drag_a
  Goto Tag Visibility7 : GotoTagVisibility  GotoTag=veh_pwr_ascent_a
  Goto Tag Visibility8 : GotoTagVisibility  GotoTag=veh_pwr_rr_a
  Goto Tag Visibility9 : GotoTagVisibility  GotoTag=wh_trq_a
  "slip, braking, traction calcs" : Subsystem
      settings: RTWFcnNameOpts=Auto  RTWFileNameOpts=Auto
  vehicle <veh> : Subsystem
      settings: RTWFcnNameOpts=Auto  RTWFileNameOpts=Auto
      mask Display: image(imread('bdi_veh.jpg'))
  wheel and axle  front/rear <wh> : Subsystem
      settings: RTWFcnNameOpts=Auto  RTWFileNameOpts=Auto
      mask Display: image(imread('bdi_wh.jpg'))
  requested out : Outport  Port=1  InitialOutput=0
  torque and speed req'd from drivetrain into front axle (Nm),(rad/s) : Outport  Port=2  InitialOutput=0
  torque and speed req'd from drivetrain into rear axle (Nm),(rad/s) : Outport  Port=3  InitialOutput=0
  sensors : Outport  Port=4  InitialOutput=0
  tag scope: current_veh_mass=scoped, grade=scoped, v_init=scoped
  wires:
  vehicle speed req'd at end of time step (m/s)/1 -> vehicle <veh>/1(vehicle speed req'd at end of time step (m/s)), Bus Creator1/1  "veh_spd_r"
  vehicle <veh>/1("tractive force and speed required of tire and wheel (N), (m/s)") -> wheel and axle  front/rear <wh>/1("tractive force and speed req'd of tire/road interface (N), (m/s)")
  wheel and axle  front/rear <wh>/3(tractive force and linear speed  achievable) -> vehicle <veh>/2(tractive force and linear speed achievable (N))
  "torque and speed available from drivetrain into front axle (Nm), (rad/s)"/1 -> wheel and axle  front/rear <wh>/2("torque and speed available from drivetrain into front axle (Nm), (rad/s)")
  "torque and speed available from drivetrain into rear axle (Nm), (rad/s)"/1 -> wheel and axle  front/rear <wh>/3("torque and speed available from drivetrain into rear axle (Nm), (rad/s)")
  wheel and axle  front/rear <wh>/1(torque and speed req'd from drivetrain into front axle (Nm),(rad/s)) -> torque and speed req'd from drivetrain into front axle (Nm),(rad/s)/1
  wheel and axle  front/rear <wh>/2(torque and speed req'd from drivetrain into rear axle (Nm),(rad/s)) -> torque and speed req'd from drivetrain into rear axle (Nm),(rad/s)/1
  control/1 -> Demux/1
  Demux/1 -> [v_init]
  Demux/2 -> [current_veh_mass]
  Demux/3 -> [grade]
  [Fr] -> Bus Creator/3  "Fr"
  Bus Creator/1 -> sensors/1
  [mpha] -> Bus Creator/1  "mpha"
  [v_prev] -> Bus Creator/2  "v_prev"
  [veh_pwr_accel_a] -> Bus Creator/4  "veh_pwr_accel_a"
  [veh_pwr_drag_a] -> Bus Creator/5  "veh_pwr_drag_a"
  [veh_pwr_ascent_a] -> Bus Creator/6  "veh_pwr_ascent_a"
  [veh_pwr_rr_a] -> Bus Creator/7  "veh_pwr_rr_a"
  [wh_trq_a] -> Bus Creator/8  "wh_trq_a"
  [F_front_brake_req] -> Bus Creator/9  "F_front_brake_req"
  [F_drivetrain_ach] -> Bus Creator/10  "F_drivetrain_ach"
  [F_front_brake] -> Bus Creator/11  "F_front_brake"
  [F_rear_brake] -> Bus Creator/12  "F_rear_brake"
  [w_wheel_ach] -> Bus Creator/13  "w_wheel_ach"
  [F_rear_drivetrain_ach] -> Bus Creator/14  "F_rear_drivetrain_ach"
  [F_max_front_brake] -> Bus Creator/15  "F_max_front_brake"
  [F_max_rear_brake] -> Bus Creator/16  "F_max_rear_brake"
  [brake_limited] -> Bus Creator/17  "brake_limited"
  [veh_spd_a_rec] -> Bus Creator/18  "veh_spd_a_rec"
  [F_req] -> Bus Creator/19  "F_req"
  [v_ave_req] -> Bus Creator/20  "v_ave_req"
  [F_req_limited] -> Bus Creator/21  "F_req_limited"
  [v_req_limited] -> Bus Creator/22  "v_req_limited"
  [wt_front_axle] -> Bus Creator/23  "wt_front_axle"
  [wt_rear_axle] -> Bus Creator/24  "wt_rear_axle"
  [front_traction_ratio] -> Bus Creator/25  "front_traction_ratio"
  [slip_limited] -> Bus Creator/26  "slip_limited"
  [F_rear_brake_req] -> Bus Creator/27  "F_rear_brake_req"
  Bus Creator1/1 -> requested out/1
